simulink model "Suspensao_Ativa"  (Simulink 7.6)
settings: Solver=ode45  StartTime=0.0  StopTime=10.0  RelTol=1e-3
values from neighbouring files (symbols this model uses):
  A = [       0,       1,         0,              -1 ... (first row only)    [SETUP_SUSP_ATIVA.m]
  B = [          0,      0 ... (first row only)    [SETUP_SUSP_ATIVA.m]
  C = [eye(4) ... (first row only)    [SETUP_SUSP_ATIVA.m]
  D = [zeros(4,2);0,0;0,1/M_s]    [SETUP_SUSP_ATIVA.m]
  K = [24.66 48.87 -0.47 3.68]    [SETUP_SUSP_ATIVA.m]
libraries: simulink x1
settings Model: Creator=Reginaldo Cardoso  LastModifiedBy=Reginaldo Cardoso
settings DebuggingCC: AlgebraicLoopMsg=none  SolverPrmCheckMsg=none
settings GRTTargetCC: CombineOutputUpdateFcns=on

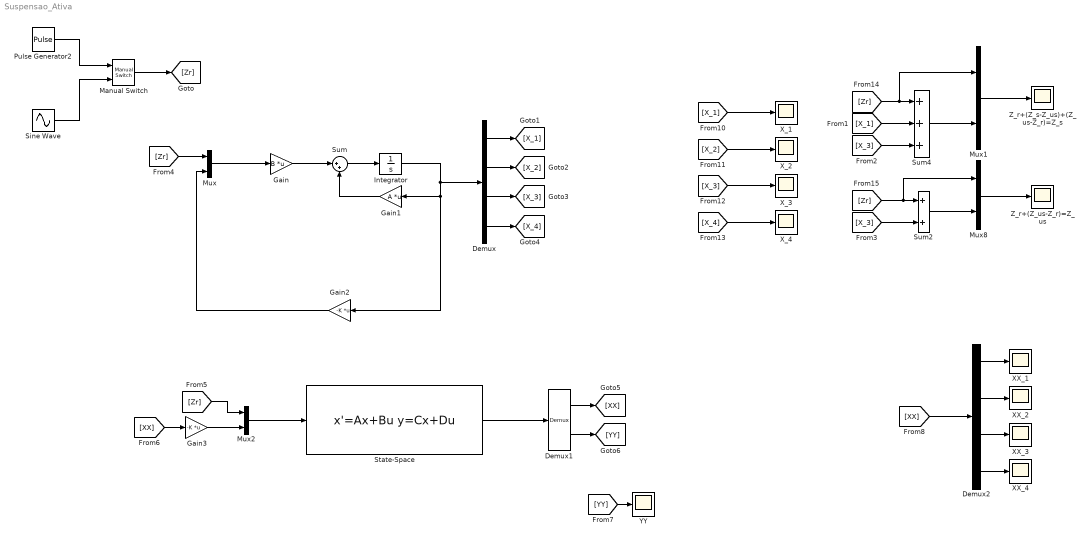
== system Suspensao_Ativa ==
  Demux : Demux
  Demux1 : Demux  Outputs=[4;2]
  Demux2 : Demux
  Gain : Gain  Gain=B  Multiplication=Matrix(K*u)
  Gain1 : Gain  Gain=A  Multiplication=Matrix(K*u)
  Gain2 : Gain  Gain=-K  Multiplication=Matrix(K*u) (u vector)
  Gain3 : Gain  Gain=-K  Multiplication=Matrix(K*u) (u vector)
  Integrator : Integrator
  Manual Switch : simulink/Signal Routing/Manual Switch  SystemSampleTime=-1  sw=1  action=0  varsize=off
  Mux{,1..2,8} (4 alike) : Mux  Inputs=2
  Pulse Generator2 : DiscretePulseGenerator  PulseType=Time based  Amplitude=0.02  Period=3  PulseWidth=50  PhaseDelay=.1
  Sine Wave : Sin  Amplitude=0.02  Frequency=pi/0.3  SampleTime=0
  State-Space : StateSpace  A=A  B=B  C=C  D=D
  Sum : Sum  Inputs=|++
  Sum2 : Sum  Inputs=2  SaturateOnIntegerOverflow=on  InputSameDT=on  OutDataTypeStr=Inherit: Same as first input
  Sum4 : Sum  Inputs=3  SaturateOnIntegerOverflow=on  InputSameDT=on  OutDataTypeStr=Inherit: Same as first input
  XX_{1..4} (4 alike) : Scope
      XX_1 settings: SaveName=x7  DataFormat=Array
      XX_2 settings: SaveName=x8  DataFormat=Array
      XX_3 settings: SaveName=x9  DataFormat=Array
      XX_4 settings: SaveName=x10  DataFormat=Array
  X_1 : Scope
      settings: SaveName=x  DataFormat=Array
  "X_2 " : Scope
      settings: SaveName=x1  DataFormat=Array
  "X_3 " : Scope
      settings: SaveName=x2  DataFormat=Array
  "X_4 " : Scope
      settings: SaveName=x3  DataFormat=Array
  YY : Scope
      settings: SaveName=x6  DataFormat=Array
  Z_r+(Z_s-Z_us)+(Z_us-Z_r)=Z_s : Scope
      settings: SaveName=x4  DataFormat=Array
  Z_r+(Z_us-Z_r)=Z_us : Scope
      settings: SaveName=x5  DataFormat=Array
  wires:
  Integrator/1 -> Gain2/1, Gain1/1, Demux/1
  Mux/1 -> Gain/1
  Gain1/1 -> Sum/2
  Gain/1 -> Sum/1
  Sum/1 -> Integrator/1
  Gain2/1 -> Mux/2
  Sine Wave/1 -> Manual Switch/2
  Pulse Generator2/1 -> Manual Switch/1
  [Zr] -> Mux1/1, Sum4/1
  [Zr] -> Sum2/1, Mux8/1
  Sum4/1 -> Mux1/2
  Sum2/1 -> Mux8/2
  Mux8/1 -> Z_r+(Z_us-Z_r)=Z_us/1
  Mux1/1 -> Z_r+(Z_s-Z_us)+(Z_us-Z_r)=Z_s/1
  Demux/1 -> [X_1]
  Demux/2 -> [X_2]
  Demux/3 -> [X_3]
  Demux/4 -> [X_4]
  [X_4] -> "X_4 "/1
  [X_3] -> "X_3 "/1
  [X_2] -> "X_2 "/1
  [X_1] -> X_1/1
  [X_1] -> Sum4/2
  [X_3] -> Sum4/3
  [X_3] -> Sum2/2
  Manual Switch/1 -> [Zr]
  [Zr] -> Mux/1
  Mux2/1 -> State-Space/1
  [Zr] -> Mux2/1
  State-Space/1 -> Demux1/1
  Gain3/1 -> Mux2/2
  Demux1/1 -> [XX]
  Demux1/2 -> [YY]
  [XX] -> Gain3/1
  [YY] -> YY/1
  [XX] -> Demux2/1
  Demux2/1 -> XX_1/1
  Demux2/2 -> XX_2/1
  Demux2/3 -> XX_3/1
  Demux2/4 -> XX_4/1
